simulink model "test"  (Simulink 7.7)
settings: Solver=ode45  StartTime=0.0  StopTime=100  FixedStep=0.01  RelTol=1e-6
PreLoadFcn:
  | aero=datcomimport('navionmodified.out');
  | load 'elevator.mat'
values from neighbouring files (symbols this model uses):
  alpha_table = [-2 0 1 2 4 8 12 16 20]    [elevator.mat]
  delCD = [0.0124 0.0108 0.0101 0.00943 0.00791 0.00435 -0.000646 -0.00885 -0.0253 0.00857 0.00726 0.00666 ... (81 elements, 9x9)]    [elevator.mat]
  delCL = [-0.228 -0.193 -0.168 -0.108 0 0.108 0.168 0.193 0.228]    [elevator.mat]
  delCm = [0.5447 0.4632 0.3984 0.2534 -0.0003 -0.2534 -0.3984 -0.4632 -0.5452]    [elevator.mat]
  delE = [-40 -30 -20 -10 0 10 20 30 40]    [elevator.mat]
undefined symbols (not defined in the file or in its folder): ft, s
libraries: aerolibasang x3, aerolib6dofsys x2, aerolibconvert2 x2, aerolibtransform2 x2, aerolibutil x1, aerolibatmos2 x1, aerolibadyn x1
settings Model: Creator=pshankar  LastModifiedBy=ggramajo
settings SolverCC: AlgebraicLoopSolver=LineSearch
settings DebuggingCC: AlgebraicLoopMsg=none  SolverPrmCheckMsg=none

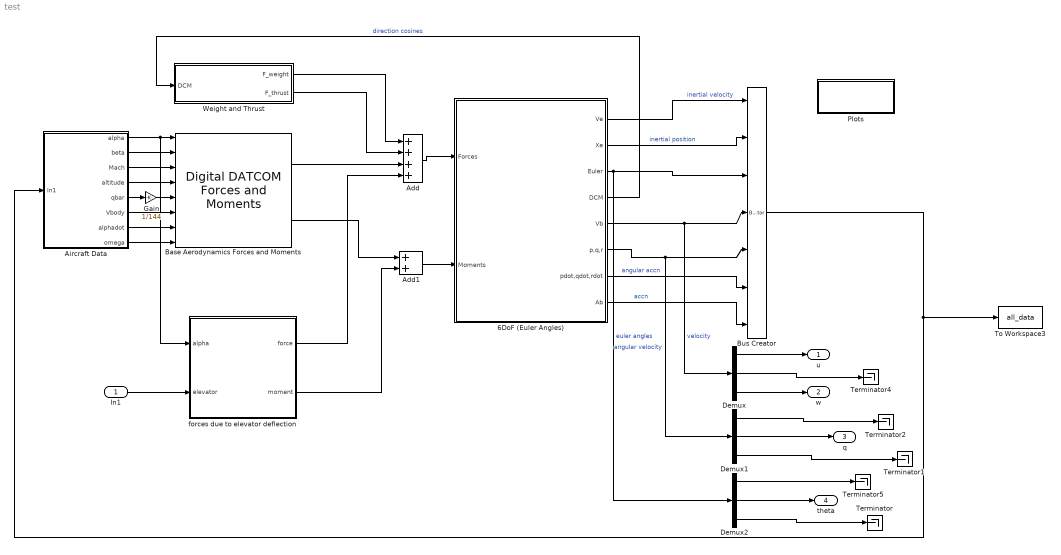
== system test ==
  In1 : Inport
  6DoF (Euler Angles) : Subsystem  AncestorBlock=aerolib6dof2/6DoF (Euler Angles)  mask(6DoF EoM (Body Axis)){units=English (Velocity in ft/s), mtype=Fixed, rep=Euler Angles, xme_0=[0 0 0], Vm_0=[175 0 0], eul_0=[0 0 0], pm_0=[0 0 0], mass_0=2750/32.2, mass_e=0.5, mass_f=2.0, inertia=[1048 0 0;0 3000 0;0 0 3530], inertia_e=eye(3), inertia_f=2*eye(3), k_quat=1.0}
      mask prompts: mtype "Mass type:"; rep "Representation:"; xme_0 "Initial position in inertial axes [Xe,Ye,Ze]:"; Vm_0 "Initial velocity in body axes [U,v,w]:"; eul_0 "Initial Euler orientation [roll, pitch, yaw]:"; pm_0 "Initial body rotation rates [p,q,r]:"; mass_0 "Initial mass:"; mass_e "Empty mass:"; mass_f "Full mass:"; inertia_e "Empty inertia matrix:"; inertia_f "Full inertia matrix:"; k_quat "Gain for quaternion normalization:"
      mask help: Integrate the six-degrees-of-freedom equations of motion in body axis.
      mask init:
      | [x y xp yp highstr lowstr maxy miny]=aeroimage('sixdofbody',gcbh);
      | ports=aeroicon('aeroblk6dofbody','icon');
      mask Help: eval('asbhelp(''sixdof_euler_angles'')');
      mask StyleString: popup(Metric (MKS)|English (Velocity in ft/s)|English (Velocity in kts)),popup(Fixed|Simple Variable|Custom Variable),popup(Euler Angles|Quaternion),edit,edit,edit,edit,edit,edit,edit,edit,edit,edit,edit
      mask CallbackString: |aeroicon('aeroblk6dofbody');|aeroicon('aeroblk6dofbody');|||||||||||
      mask Display:
      | port_label(ports(1).type,ports(1).port,ports(1).txt,'texmode','on');
      | port_label(ports(2).type,ports(2).port,ports(2).txt,'texmode','on');
      | port_label(ports(3).type,ports(3).port,ports(3).txt,'texmode','on');
      | port_label(ports(4).type,ports(4).port,ports(4).txt,'texmode','on');
      | port_label(ports(5).type,ports(5).port,ports(5).txt,'texmode','on');
      | port_label(ports(6).type,ports(6).port,ports(6).txt,'texmode','on');
      | port_label(ports(7).type,ports(7).port,ports(7).txt,'texmode','on');
      | port_label(ports(8).type,ports(8).port,ports(8).txt,'texmode','on');
      | port_label(ports(9).type,ports(9).port,ports(9).txt,'texmode','on');
      | port_label(ports(10).type,ports(10).port,ports(10).txt,'texmode','on');
      | port_label(ports(11).type,ports(11).port,ports(11).txt,'texmode','on');
      | port_label(ports(12).type,ports(12).port,ports(12).txt,'texmode','on');
      | port_label(ports(13).type,ports(13).port,ports(13).txt,'texmode','on');
      | port_label(ports(14).type,ports(14).port,ports(14).txt,'texmode','on');
      | port_label(ports(15).type,ports(15).port,ports(15).txt,'texmode','on');
      | text(0.5,maxy+0.065,highstr{:},'horizontalAlignment','center')
      | text(0.5,miny-0.05,lowstr{:},'horizontalAlignment','center')
      | plot(x,y);
      | patch(xp, yp);
  Add : Sum  Inputs=++++
  Add1 : Sum
  Aircraft Data : Subsystem
  Base Aerodynamics Forces and Moments : aerolibadyn/Digital DATCOM Forces and Moments  SystemSampleTime=-1  units=English (Velocity in ft/s)  dcase=aero{1}  fmode=Body  buildno=0  imethod=Linear  emethod=Linear  rmethod=Linear Extrapolation  action=None
  Bus Creator : BusCreator  Inputs=7
  Demux : Demux  Outputs=3
  Demux1 : Demux  Outputs=3
  Demux2 : Demux  Outputs=3
  Gain : Gain  Gain=1/144
  Plots : Subsystem  TreatAsAtomicUnit=on
      settings: OpenFcn=plotdata_Gramajo
  Terminator{,1..2,4..5} (5 alike) : Terminator
  To Workspace3 : ToWorkspace  VariableName=all_data  SampleTime=-1  SaveFormat=Array
  Weight and Thrust : Subsystem
  forces due to elevator deflection : Subsystem
  u : Outport
  w : Outport  Port=2
  q : Outport  Port=3
  theta : Outport  Port=4
  wires:
  6DoF (Euler Angles)/1(Ve) -> Bus Creator/1  "inertial velocity"
  6DoF (Euler Angles)/2(Xe) -> Bus Creator/2  "inertial position"
  6DoF (Euler Angles)/3(Euler) -> Bus Creator/3, Demux2/1  "euler angles"
  6DoF (Euler Angles)/6(p,q,r) -> Bus Creator/5, Demux1/1  "angular velocity"
  Bus Creator/1 -> Aircraft Data/1(In1), To Workspace3/1
  6DoF (Euler Angles)/5(Vb) -> Bus Creator/4, Demux/1  "velocity"
  6DoF (Euler Angles)/7(pdot,qdot,rdot) -> Bus Creator/6  "angular accn"
  6DoF (Euler Angles)/8(Ab) -> Bus Creator/7  "accn"
  Add/1 -> 6DoF (Euler Angles)/1(Forces)
  Weight and Thrust/1(F_weight) -> Add/1
  6DoF (Euler Angles)/4(DCM) -> Weight and Thrust/1(DCM)  "direction cosines"
  Aircraft Data/1(alpha) -> Base Aerodynamics Forces and Moments/1, forces due to elevator deflection/1(alpha)
  Aircraft Data/2(beta) -> Base Aerodynamics Forces and Moments/2
  Aircraft Data/3(Mach) -> Base Aerodynamics Forces and Moments/3
  Aircraft Data/4(altitude) -> Base Aerodynamics Forces and Moments/4
  Aircraft Data/5(qbar) -> Gain/1
  Aircraft Data/6(Vbody) -> Base Aerodynamics Forces and Moments/6
  Aircraft Data/7(alphadot) -> Base Aerodynamics Forces and Moments/7
  Aircraft Data/8(omega) -> Base Aerodynamics Forces and Moments/8
  Weight and Thrust/2(F_thrust) -> Add/2
  Base Aerodynamics Forces and Moments/1 -> Add/3
  Base Aerodynamics Forces and Moments/2 -> Add1/1
  Gain/1 -> Base Aerodynamics Forces and Moments/5
  Add1/1 -> 6DoF (Euler Angles)/2(Moments)
  forces due to elevator deflection/1(force) -> Add/4
  forces due to elevator deflection/2(moment) -> Add1/2
  In1/1 -> forces due to elevator deflection/2(elevator)
  Demux2/2 -> theta/1
  Demux/1 -> u/1
  Demux/3 -> w/1
  Demux/2 -> Terminator4/1
  Demux2/1 -> Terminator5/1
  Demux2/3 -> Terminator/1
  Demux1/2 -> q/1
  Demux1/1 -> Terminator2/1
  Demux1/3 -> Terminator1/1

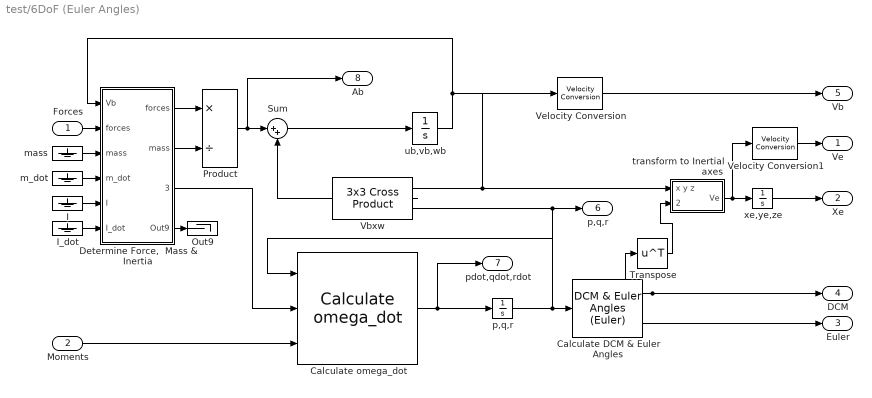
== system test/6DoF (Euler Angles) ==
  Forces : Inport
  Moments : Inport  Port=2
  Calculate DCM & Euler Angles : aerolib6dofsys/DCM & Euler Angles (Euler)  SystemSampleTime=-1
  Calculate omega_dot : aerolib6dofsys/Calculate omega_dot  SystemSampleTime=-1
  "Determine Force,  Mass & Inertia" : Subsystem  AncestorBlock=aerolib6dofsys/Mass & Inertia (fixed)
      mask Type: Mass & Inertia (fixed)
  I : Ground
  I_dot : Ground
  Out9 : Terminator
  Product : Product  Inputs=*/  SaturateOnIntegerOverflow=on  OutDataTypeStr=Inherit: Same as first input
  Sum : Sum  Inputs=|++  SaturateOnIntegerOverflow=on
  Transpose : Math  Operator=transpose  SaturateOnIntegerOverflow=on
  Vbxw : aerolibutil/3x3 Cross Product  SystemSampleTime=-1
  Velocity Conversion : aerolibconvert2/Velocity Conversion  SystemSampleTime=-1  IU=ft/s  OU=ft/s
  Velocity Conversion1 : aerolibconvert2/Velocity Conversion  SystemSampleTime=-1  IU=ft/s  OU=ft/s
  m_dot : Ground
  mass : Ground
  "p,q,r " : Integrator  InitialCondition=pm_0
  "transform to Inertial axes " : Subsystem
      mask Type: Vector Transformation
      mask Display: disp('L_EB')
  ub,vb,wb : Integrator  InitialCondition=convvel(Vm_0,'ft/s','ft/s')
  xe,ye,ze : Integrator  InitialCondition=xme_0
  Ve : Outport
  Xe : Outport  Port=2
  Euler : Outport  Port=3
  DCM : Outport  Port=4
  Vb : Outport  Port=5
  p,q,r : Outport  Port=6
  pdot,qdot,rdot : Outport  Port=7
  Ab : Outport  Port=8
  wires:
  "Determine Force,  Mass & Inertia"/1("forces ") -> Product/1
  I_dot/1 -> "Determine Force,  Mass & Inertia"/6(I_dot)
  I/1 -> "Determine Force,  Mass & Inertia"/5(I)
  Calculate omega_dot/1 -> "p,q,r "/1, pdot,qdot,rdot/1
  "Determine Force,  Mass & Inertia"/4(Out9) -> Out9/1
  m_dot/1 -> "Determine Force,  Mass & Inertia"/4(m_dot)
  "Determine Force,  Mass & Inertia"/2(mass) -> Product/2
  mass/1 -> "Determine Force,  Mass & Inertia"/3("mass ")
  Transpose/1 -> "transform to Inertial axes "/2(transform coefficients)
  Calculate DCM & Euler Angles/1 -> Transpose/1, DCM/1
  Product/1 -> Ab/1, Sum/1
  Forces/1 -> "Determine Force,  Mass & Inertia"/2(forces)
  Moments/1 -> Calculate omega_dot/3
  "p,q,r "/1 -> Calculate omega_dot/1, Calculate DCM & Euler Angles/1, Vbxw/2, p,q,r/1
  "transform to Inertial axes "/1(Ve) -> xe,ye,ze/1, Velocity Conversion1/1
  xe,ye,ze/1 -> Xe/1
  Sum/1 -> ub,vb,wb/1
  ub,vb,wb/1 -> "Determine Force,  Mass & Inertia"/1(Vb), Vbxw/1, "transform to Inertial axes "/1(x y z), Velocity Conversion/1
  Vbxw/1 -> Sum/2
  Calculate DCM & Euler Angles/2 -> Euler/1
  "Determine Force,  Mass & Inertia"/3("inertia, 0") -> Calculate omega_dot/2
  Velocity Conversion/1 -> Vb/1
  Velocity Conversion1/1 -> Ve/1

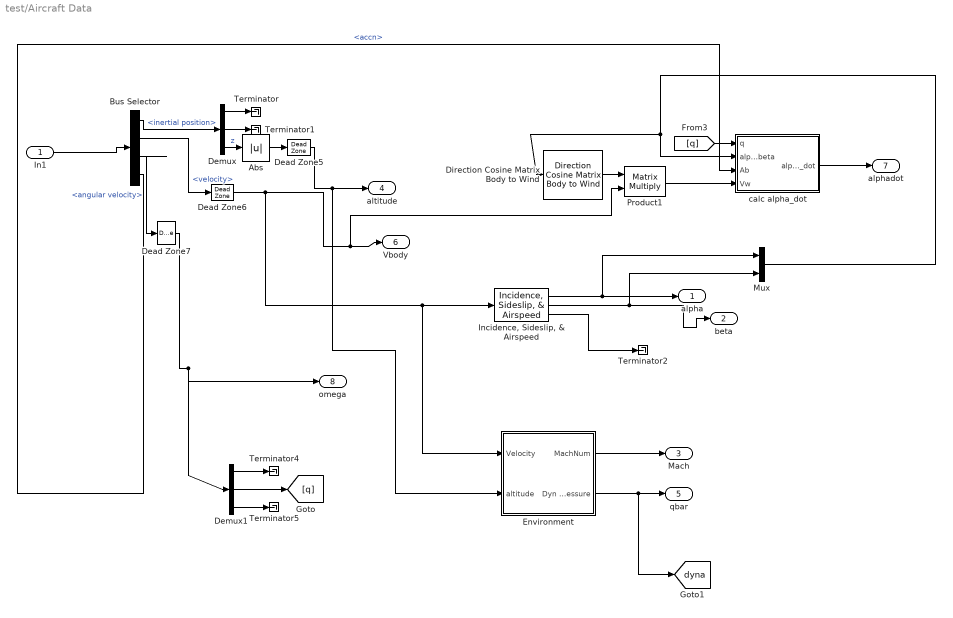
== system test/Aircraft Data ==
  In1 : Inport
  Abs : Abs
  Bus Selector : BusSelector  OutputSignals=inertial position,velocity,angular velocity,accn
  Dead Zone5 : DeadZone  LowerValue=-1e-3  UpperValue=+1e-3  SaturateOnIntegerOverflow=on
  Dead Zone6 : DeadZone  LowerValue=-1e-3  UpperValue=+1e-3  SaturateOnIntegerOverflow=on
  Dead Zone7 : DeadZone  LowerValue=-1e-3  UpperValue=+1e-3  SaturateOnIntegerOverflow=on
  Demux : Demux  Outputs=3
  Demux1 : Demux  Outputs=3
  Direction Cosine Matrix Body to Wind : aerolibtransform2/Direction Cosine Matrix Body to Wind  SystemSampleTime=-1
  Environment : Subsystem
  "Incidence, Sideslip, & Airspeed" : aerolibasang/Incidence, Sideslip, & Airspeed  SystemSampleTime=-1
  Mux : Mux  Inputs=2
  Product1 : Product  Multiplication=Matrix(*)  SaturateOnIntegerOverflow=on  InputSameDT=on  OutDataTypeStr=Inherit: Same as first input
  Terminator{,1..2,4..5} (5 alike) : Terminator
  calc alpha_dot : Subsystem
  alpha : Outport
  beta : Outport  Port=2
  Mach : Outport  Port=3
  altitude : Outport  Port=4
  qbar : Outport  Port=5
  Vbody : Outport  Port=6
  alphadot : Outport  Port=7
  omega : Outport  Port=8
  tag scope: dyna=global
  wires:
  In1/1 -> Bus Selector/1
  Bus Selector/2 -> Dead Zone6/1  "<velocity>"
  Bus Selector/1 -> Demux/1  "<inertial position>"
  Demux/3 -> Abs/1  "z"
  Bus Selector/3 -> Dead Zone7/1  "<angular velocity>"
  Demux/1 -> Terminator/1
  Demux/2 -> Terminator1/1
  Abs/1 -> Dead Zone5/1
  Dead Zone5/1 -> altitude/1, Environment/2(altitude)
  Dead Zone6/1 -> Vbody/1, Product1/2, "Incidence, Sideslip, & Airspeed"/1, Environment/1(Velocity)
  Dead Zone7/1 -> omega/1, Demux1/1
  "Incidence, Sideslip, & Airspeed"/1 -> alpha/1, Mux/1
  "Incidence, Sideslip, & Airspeed"/2 -> beta/1, Mux/2
  "Incidence, Sideslip, & Airspeed"/3 -> Terminator2/1
  calc alpha_dot/1(alpha_dot) -> alphadot/1
  [q] -> calc alpha_dot/1(q)
  Direction Cosine Matrix Body to Wind/1 -> Product1/1
  Product1/1 -> calc alpha_dot/4(Vw)
  Bus Selector/4 -> calc alpha_dot/3(Ab)  "<accn>"
  Mux/1 -> calc alpha_dot/2(alpha,beta), Direction Cosine Matrix Body to Wind/1
  Environment/1(MachNum) -> Mach/1
  Environment/2(Dyn Pressure) -> qbar/1, [dyna]
  Demux1/3 -> Terminator5/1
  Demux1/1 -> Terminator4/1
  Demux1/2 -> [q]

== system test/Plots ==

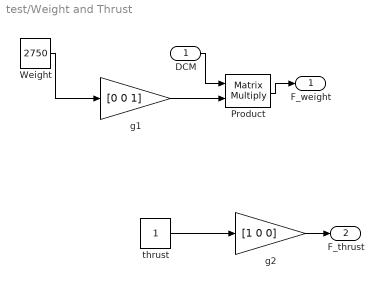
== system test/Weight and Thrust ==
  DCM : Inport
  Product : Product  Multiplication=Matrix(*)  SaturateOnIntegerOverflow=on  InputSameDT=on  OutDataTypeStr=Inherit: Same as first input
  Weight : Constant  Value=2750
  g1 : Gain  Gain=[0 0 1]  SaturateOnIntegerOverflow=on  OutDataTypeStr=Inherit: Same as input  ParamDataTypeStr=Inherit: Same as input
  g2 : Gain  Gain=[1 0 0]  SaturateOnIntegerOverflow=on  OutDataTypeStr=Inherit: Same as input  ParamDataTypeStr=Inherit: Same as input
  thrust : Constant
  F_weight : Outport
  F_thrust : Outport  Port=2
  wires:
  thrust/1 -> g2/1
  Weight/1 -> g1/1
  DCM/1 -> Product/1
  Product/1 -> F_weight/1
  g2/1 -> F_thrust/1
  g1/1 -> Product/2

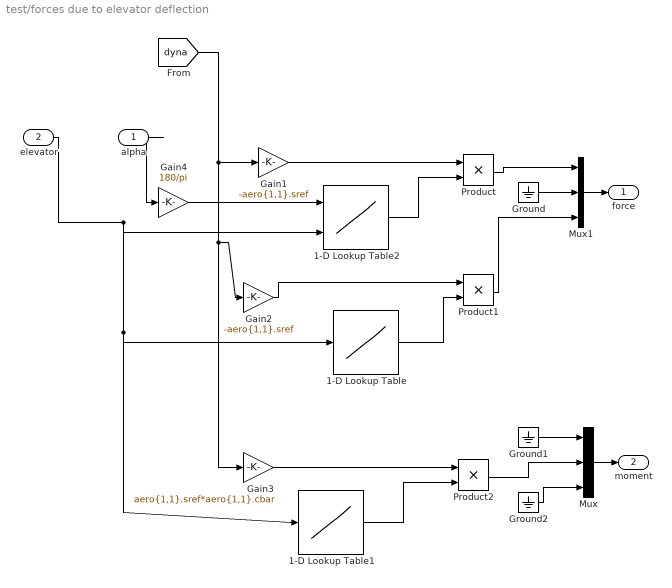
== system test/forces due to elevator deflection ==
  alpha : Inport
  elevator : Inport  Port=2
  1-D Lookup Table : Lookup_n-D  NumberOfTableDimensions=1  BreakpointsForDimension1=delE  Table=delCL  RndMeth=Simplest  InputSameDT=on
  1-D Lookup Table1 : Lookup_n-D  NumberOfTableDimensions=1  BreakpointsForDimension1=delE  Table=delCm  RndMeth=Simplest  InputSameDT=on
  1-D Lookup Table2 : Lookup_n-D  BreakpointsForDimension1=alpha_table  BreakpointsForDimension2=delE  Table=delCD  RndMeth=Simplest  InputSameDT=on
  Gain1 : Gain  Gain=-aero{1,1}.sref
  Gain2 : Gain  Gain=-aero{1,1}.sref
  Gain3 : Gain  Gain=aero{1,1}.sref*aero{1,1}.cbar
  Gain4 : Gain  Gain=180/pi
  Ground : Ground
  Ground1 : Ground
  Ground2 : Ground
  Mux : Mux  Inputs=3
  Mux1 : Mux  Inputs=3
  Product : Product  RndMeth=Zero
  Product1 : Product  RndMeth=Zero
  Product2 : Product  RndMeth=Zero
  force : Outport
  moment : Outport  Port=2
  wires:
  Ground/1 -> Mux1/2
  Ground1/1 -> Mux/1
  Ground2/1 -> Mux/3
  Product/1 -> Mux1/1
  Product1/1 -> Mux1/3
  Gain1/1 -> Product/1
  Gain2/1 -> Product1/1
  Product2/1 -> Mux/2
  Gain3/1 -> Product2/1
  [dyna] -> Gain3/1, Gain2/1, Gain1/1
  Mux1/1 -> force/1
  1-D Lookup Table/1 -> Product1/2
  Mux/1 -> moment/1
  1-D Lookup Table1/1 -> Product2/2
  elevator/1 -> 1-D Lookup Table2/2, 1-D Lookup Table/1, 1-D Lookup Table1/1
  alpha/1 -> Gain4/1
  Gain4/1 -> 1-D Lookup Table2/1
  1-D Lookup Table2/1 -> Product/2

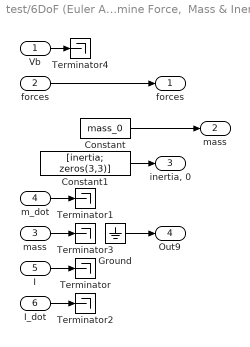
== system test/6DoF (Euler Angles)/Determine Force,  Mass & Inertia ==
  Vb : Inport
  forces : Inport  Port=2
  "mass " : Inport  Port=3
  m_dot : Inport  Port=4  OutDataTypeStr=double
  I : Inport  Port=5  OutDataTypeStr=double
  I_dot : Inport  Port=6  OutDataTypeStr=double
  Constant : Constant  Value=mass_0  OutDataTypeStr=Inherit: Inherit via back propagation
  Constant1 : Constant  Value=[inertia; zeros(3,3)]  OutDataTypeStr=Inherit: Inherit via back propagation
  Ground : Ground
  Terminator{,1..4} (5 alike) : Terminator
  "forces " : Outport
  mass : Outport  Port=2
  "inertia, 0" : Outport  Port=3
  Out9 : Outport  Port=4
  wires:
  Vb/1 -> Terminator4/1
  forces/1 -> "forces "/1
  "mass "/1 -> Terminator3/1
  I_dot/1 -> Terminator2/1
  m_dot/1 -> Terminator1/1
  I/1 -> Terminator/1
  Ground/1 -> Out9/1
  Constant1/1 -> "inertia, 0"/1
  Constant/1 -> mass/1

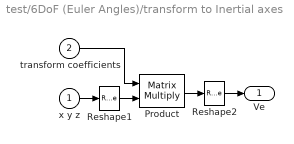
== system test/6DoF (Euler Angles)/transform to Inertial axes  ==
  x y z : Inport
  transform coefficients : Inport  Port=2
  Product : Product  Multiplication=Matrix(*)  SaturateOnIntegerOverflow=on  InputSameDT=on  OutDataTypeStr=Inherit: Same as first input
  Reshape1 : Reshape  OutputDimensionality=Column vector (2-D)
  Reshape2 : Reshape
  Ve : Outport
  wires:
  Reshape2/1 -> Ve/1
  Reshape1/1 -> Product/2
  x y z/1 -> Reshape1/1
  transform coefficients/1 -> Product/1
  Product/1 -> Reshape2/1

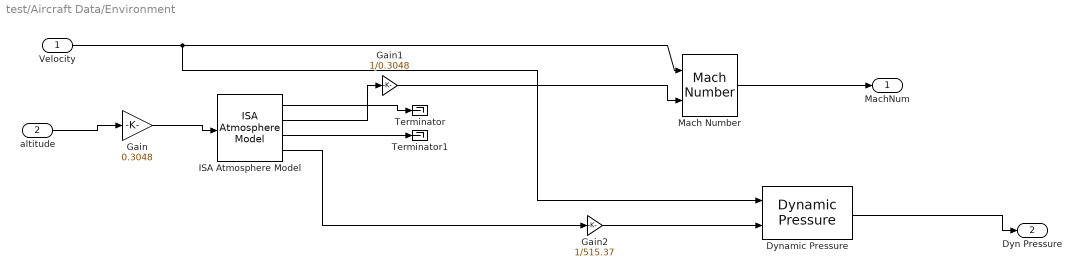
== system test/Aircraft Data/Environment ==
  Velocity : Inport
  altitude : Inport  Port=2
  Dynamic Pressure : aerolibasang/Dynamic Pressure  SystemSampleTime=-1
  Gain : Gain  Gain=0.3048
  Gain1 : Gain  Gain=1/0.3048
  Gain2 : Gain  Gain=1/515.37
  ISA Atmosphere Model : aerolibatmos2/ISA Atmosphere Model  SystemSampleTime=-1  custom=off  g=9.80665  gamma=1.4  R=287.0531  L=0.0065  h_trop=11000  h_strat=20000  rho0=1.225  P0=101325  T0=288.15
  Mach Number : aerolibasang/Mach Number  SystemSampleTime=-1
  Terminator : Terminator
  Terminator1 : Terminator
  MachNum : Outport
  Dyn Pressure : Outport  Port=2
  wires:
  ISA Atmosphere Model/1 -> Terminator/1
  ISA Atmosphere Model/3 -> Terminator1/1
  ISA Atmosphere Model/2 -> Gain1/1
  Gain1/1 -> Mach Number/2
  ISA Atmosphere Model/4 -> Gain2/1
  Gain2/1 -> Dynamic Pressure/2
  Velocity/1 -> Mach Number/1, Dynamic Pressure/1
  altitude/1 -> Gain/1
  Mach Number/1 -> MachNum/1
  Dynamic Pressure/1 -> Dyn Pressure/1
  Gain/1 -> ISA Atmosphere Model/1

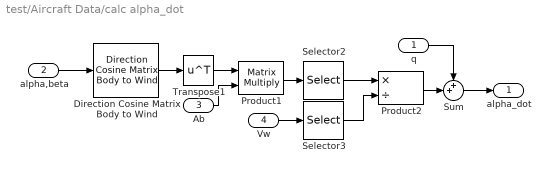
== system test/Aircraft Data/calc alpha_dot ==
  q : Inport
  alpha,beta : Inport  Port=2
  Ab : Inport  Port=3
  Vw : Inport  Port=4
  Direction Cosine Matrix Body to Wind : aerolibtransform2/Direction Cosine Matrix Body to Wind  SystemSampleTime=-1
  Product1 : Product  Multiplication=Matrix(*)  SaturateOnIntegerOverflow=on  InputSameDT=on  OutDataTypeStr=Inherit: Same as first input
  Product2 : Product  Inputs=*/  SaturateOnIntegerOverflow=on  InputSameDT=on  OutDataTypeStr=Inherit: Same as first input
  Selector2 : Selector  InputPortWidth=3  IndexOptions=Index vector (dialog)  Indices=3  OutputSizes=1
  Selector3 : Selector  InputPortWidth=3  IndexOptions=Index vector (dialog)  Indices=1  OutputSizes=1
  Sum : Sum  Inputs=++|
  Transpose1 : Math  Operator=transpose  SaturateOnIntegerOverflow=on
  alpha_dot : Outport
  wires:
  Direction Cosine Matrix Body to Wind/1 -> Transpose1/1
  Transpose1/1 -> Product1/1
  Product1/1 -> Selector2/1
  Selector2/1 -> Product2/1
  Selector3/1 -> Product2/2
  Product2/1 -> Sum/2
  alpha,beta/1 -> Direction Cosine Matrix Body to Wind/1
  q/1 -> Sum/1
  Sum/1 -> alpha_dot/1
  Ab/1 -> Product1/2
  Vw/1 -> Selector3/1
